simulink model "CAR_CONTROL_SYSTEM"  (R2024b)
settings: Solver=FixedStepAuto  StartTime=0.0  StopTime=inf  FixedStep=1e-3  RelTol=1e-3  EnableMultiTasking=on
model workspace (MAT data in the model file):
  SL_ROS_VariableLengthArrays_MaxSizes : object (value not decoded)
undefined symbols (not defined in the file or in its folder): angular, CIRCUIT, CLTF_DAMP, CLTF_FREQ, CLTF_GAIN, CONTROL, CONTROL_INI, DiscIntNeverNeededParam, dspblkCoreblockFVToolHelper, gcbh, INPUT, linear, MCP3201, MD25, MODEL, MODEL_INI, mpcstate, MPU60X0, MPU9250, MSG, NAV_MPC_CONTROL, OUTPUT, SAMPLING_TIME, SYSID_INPUT, VL6180X
libraries: raspberrypiCommlib x153, simulink x85, raspberrypiNetworklib x8, embedlinuxBasiclib x6, ctrlSharedLib x2, ros2lib x2, mpclib x1, vrlib x1, sldrtlib x1
(part 6 of 16)

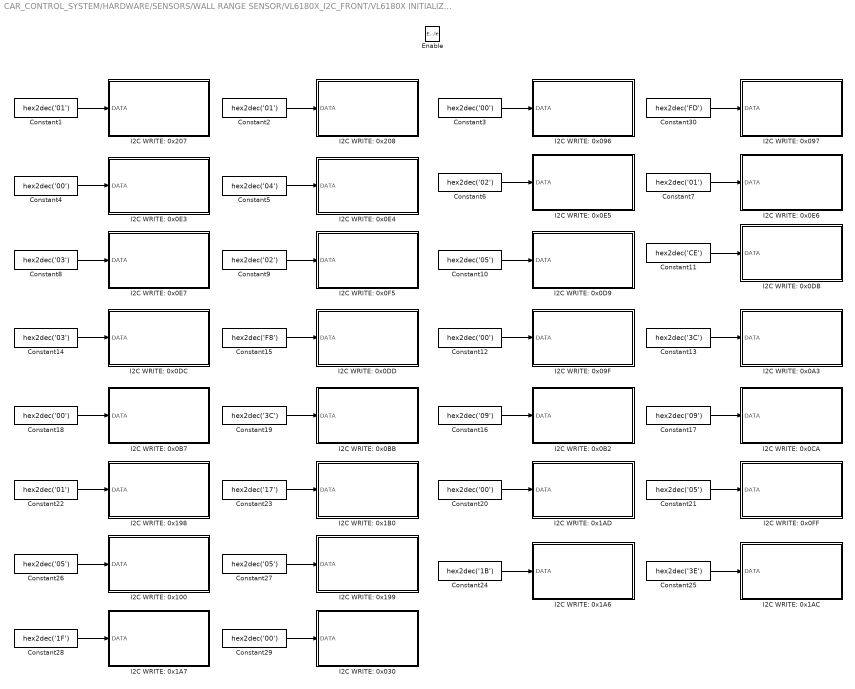
== system CAR_CONTROL_SYSTEM/HARDWARE/SENSORS/WALL RANGE SENSOR/VL6180X_I2C_FRONT/VL6180X INITIALIZATION/LOAD PRIVATE REGISTERS (MANDATORY) ==
  Enable : EnablePort
  Constant{1..2,7,22} (4 alike) : Constant  Value=hex2dec('01')  OutDataTypeStr=uint8  SampleTime=SAMPLING_TIME
  Constant{10,21,26..27} (4 alike) : Constant  Value=hex2dec('05')  OutDataTypeStr=uint8  SampleTime=SAMPLING_TIME
  Constant11 : Constant  Value=hex2dec('CE')  OutDataTypeStr=uint8  SampleTime=SAMPLING_TIME
  Constant{3..4,12,18,20,29} (6 alike) : Constant  Value=hex2dec('00')  OutDataTypeStr=uint8  SampleTime=SAMPLING_TIME
  Constant13 : Constant  Value=hex2dec('3C')  OutDataTypeStr=uint8  SampleTime=SAMPLING_TIME
  Constant14 : Constant  Value=hex2dec('03')  OutDataTypeStr=uint8  SampleTime=SAMPLING_TIME
  Constant15 : Constant  Value=hex2dec('F8')  OutDataTypeStr=uint8  SampleTime=SAMPLING_TIME
  Constant16 : Constant  Value=hex2dec('09')  OutDataTypeStr=uint8  SampleTime=SAMPLING_TIME
  Constant17 : Constant  Value=hex2dec('09')  OutDataTypeStr=uint8  SampleTime=SAMPLING_TIME
  Constant19 : Constant  Value=hex2dec('3C')  OutDataTypeStr=uint8  SampleTime=SAMPLING_TIME
  Constant23 : Constant  Value=hex2dec('17')  OutDataTypeStr=uint8  SampleTime=SAMPLING_TIME
  Constant24 : Constant  Value=hex2dec('1B')  OutDataTypeStr=uint8  SampleTime=SAMPLING_TIME
  Constant25 : Constant  Value=hex2dec('3E')  OutDataTypeStr=uint8  SampleTime=SAMPLING_TIME
  Constant28 : Constant  Value=hex2dec('1F')  OutDataTypeStr=uint8  SampleTime=SAMPLING_TIME
  Constant30 : Constant  Value=hex2dec('FD')  OutDataTypeStr=uint8  SampleTime=SAMPLING_TIME
  Constant5 : Constant  Value=hex2dec('04')  OutDataTypeStr=uint8  SampleTime=SAMPLING_TIME
  Constant6 : Constant  Value=hex2dec('02')  OutDataTypeStr=uint8  SampleTime=SAMPLING_TIME
  Constant8 : Constant  Value=hex2dec('03')  OutDataTypeStr=uint8  SampleTime=SAMPLING_TIME
  Constant9 : Constant  Value=hex2dec('02')  OutDataTypeStr=uint8  SampleTime=SAMPLING_TIME
  "I2C WRITE: 0x030 " : Subsystem  mask{SLAVE_ADDRESS=VL6180X.ADDRESS, REGISTER_ADDRESS=hex2dec('030')}
      mask prompts: SLAVE_ADDRESS "SLAVE ADDRESS"; REGISTER_ADDRESS "REGISTER ADDRESS"
      mask init:
      | REGISTER_ADDRESS_MSB = uint8(floor(REGISTER_ADDRESS/(2^8)));
      | REGISTER_ADDRESS_LSB = uint8(rem(REGISTER_ADDRESS,2^8));
  I2C WRITE: 0x096 : Subsystem  mask{SLAVE_ADDRESS=VL6180X.ADDRESS, REGISTER_ADDRESS=hex2dec('096')}
      mask prompts: SLAVE_ADDRESS "SLAVE ADDRESS"; REGISTER_ADDRESS "REGISTER ADDRESS"
      mask init:
      | REGISTER_ADDRESS_MSB = uint8(floor(REGISTER_ADDRESS/(2^8)));
      | REGISTER_ADDRESS_LSB = uint8(rem(REGISTER_ADDRESS,2^8));
  I2C WRITE: 0x097 : Subsystem  mask{SLAVE_ADDRESS=VL6180X.ADDRESS, REGISTER_ADDRESS=hex2dec('097')}
      mask prompts: SLAVE_ADDRESS "SLAVE ADDRESS"; REGISTER_ADDRESS "REGISTER ADDRESS"
      mask init:
      | REGISTER_ADDRESS_MSB = uint8(floor(REGISTER_ADDRESS/(2^8)));
      | REGISTER_ADDRESS_LSB = uint8(rem(REGISTER_ADDRESS,2^8));
  I2C WRITE: 0x09F : Subsystem  mask{SLAVE_ADDRESS=VL6180X.ADDRESS, REGISTER_ADDRESS=hex2dec('09F')}
      mask prompts: SLAVE_ADDRESS "SLAVE ADDRESS"; REGISTER_ADDRESS "REGISTER ADDRESS"
      mask init:
      | REGISTER_ADDRESS_MSB = uint8(floor(REGISTER_ADDRESS/(2^8)));
      | REGISTER_ADDRESS_LSB = uint8(rem(REGISTER_ADDRESS,2^8));
  I2C WRITE: 0x0A3 : Subsystem  mask{SLAVE_ADDRESS=VL6180X.ADDRESS, REGISTER_ADDRESS=hex2dec('0A3')}
      mask prompts: SLAVE_ADDRESS "SLAVE ADDRESS"; REGISTER_ADDRESS "REGISTER ADDRESS"
      mask init:
      | REGISTER_ADDRESS_MSB = uint8(floor(REGISTER_ADDRESS/(2^8)));
      | REGISTER_ADDRESS_LSB = uint8(rem(REGISTER_ADDRESS,2^8));
  I2C WRITE: 0x0B2 : Subsystem  mask{SLAVE_ADDRESS=VL6180X.ADDRESS, REGISTER_ADDRESS=hex2dec('0B2')}
      mask prompts: SLAVE_ADDRESS "SLAVE ADDRESS"; REGISTER_ADDRESS "REGISTER ADDRESS"
      mask init:
      | REGISTER_ADDRESS_MSB = uint8(floor(REGISTER_ADDRESS/(2^8)));
      | REGISTER_ADDRESS_LSB = uint8(rem(REGISTER_ADDRESS,2^8));
  I2C WRITE: 0x0B7 : Subsystem  mask{SLAVE_ADDRESS=VL6180X.ADDRESS, REGISTER_ADDRESS=hex2dec('0B7')}
      mask prompts: SLAVE_ADDRESS "SLAVE ADDRESS"; REGISTER_ADDRESS "REGISTER ADDRESS"
      mask init:
      | REGISTER_ADDRESS_MSB = uint8(floor(REGISTER_ADDRESS/(2^8)));
      | REGISTER_ADDRESS_LSB = uint8(rem(REGISTER_ADDRESS,2^8));
  I2C WRITE: 0x0BB : Subsystem  mask{SLAVE_ADDRESS=VL6180X.ADDRESS, REGISTER_ADDRESS=hex2dec('0BB')}
      mask prompts: SLAVE_ADDRESS "SLAVE ADDRESS"; REGISTER_ADDRESS "REGISTER ADDRESS"
      mask init:
      | REGISTER_ADDRESS_MSB = uint8(floor(REGISTER_ADDRESS/(2^8)));
      | REGISTER_ADDRESS_LSB = uint8(rem(REGISTER_ADDRESS,2^8));
  I2C WRITE: 0x0CA : Subsystem  mask{SLAVE_ADDRESS=VL6180X.ADDRESS, REGISTER_ADDRESS=hex2dec('0CA')}
      mask prompts: SLAVE_ADDRESS "SLAVE ADDRESS"; REGISTER_ADDRESS "REGISTER ADDRESS"
      mask init:
      | REGISTER_ADDRESS_MSB = uint8(floor(REGISTER_ADDRESS/(2^8)));
      | REGISTER_ADDRESS_LSB = uint8(rem(REGISTER_ADDRESS,2^8));
  I2C WRITE: 0x0D9 : Subsystem  mask{SLAVE_ADDRESS=VL6180X.ADDRESS, REGISTER_ADDRESS=hex2dec('0D9')}
      mask prompts: SLAVE_ADDRESS "SLAVE ADDRESS"; REGISTER_ADDRESS "REGISTER ADDRESS"
      mask init:
      | REGISTER_ADDRESS_MSB = uint8(floor(REGISTER_ADDRESS/(2^8)));
      | REGISTER_ADDRESS_LSB = uint8(rem(REGISTER_ADDRESS,2^8));
  I2C WRITE: 0x0DB : Subsystem  mask{SLAVE_ADDRESS=VL6180X.ADDRESS, REGISTER_ADDRESS=hex2dec('0DB')}
      mask prompts: SLAVE_ADDRESS "SLAVE ADDRESS"; REGISTER_ADDRESS "REGISTER ADDRESS"
      mask init:
      | REGISTER_ADDRESS_MSB = uint8(floor(REGISTER_ADDRESS/(2^8)));
      | REGISTER_ADDRESS_LSB = uint8(rem(REGISTER_ADDRESS,2^8));
  I2C WRITE: 0x0DC : Subsystem  mask{SLAVE_ADDRESS=VL6180X.ADDRESS, REGISTER_ADDRESS=hex2dec('0DB')}
      mask prompts: SLAVE_ADDRESS "SLAVE ADDRESS"; REGISTER_ADDRESS "REGISTER ADDRESS"
      mask init:
      | REGISTER_ADDRESS_MSB = uint8(floor(REGISTER_ADDRESS/(2^8)));
      | REGISTER_ADDRESS_LSB = uint8(rem(REGISTER_ADDRESS,2^8));
  I2C WRITE: 0x0DD : Subsystem  mask{SLAVE_ADDRESS=VL6180X.ADDRESS, REGISTER_ADDRESS=hex2dec('0DD')}
      mask prompts: SLAVE_ADDRESS "SLAVE ADDRESS"; REGISTER_ADDRESS "REGISTER ADDRESS"
      mask init:
      | REGISTER_ADDRESS_MSB = uint8(floor(REGISTER_ADDRESS/(2^8)));
      | REGISTER_ADDRESS_LSB = uint8(rem(REGISTER_ADDRESS,2^8));
  I2C WRITE: 0x0E3 : Subsystem  mask{SLAVE_ADDRESS=VL6180X.ADDRESS, REGISTER_ADDRESS=hex2dec('0E3')}
      mask prompts: SLAVE_ADDRESS "SLAVE ADDRESS"; REGISTER_ADDRESS "REGISTER ADDRESS"
      mask init:
      | REGISTER_ADDRESS_MSB = uint8(floor(REGISTER_ADDRESS/(2^8)));
      | REGISTER_ADDRESS_LSB = uint8(rem(REGISTER_ADDRESS,2^8));
  I2C WRITE: 0x0E4 : Subsystem  mask{SLAVE_ADDRESS=VL6180X.ADDRESS, REGISTER_ADDRESS=hex2dec('0E4')}
      mask prompts: SLAVE_ADDRESS "SLAVE ADDRESS"; REGISTER_ADDRESS "REGISTER ADDRESS"
      mask init:
      | REGISTER_ADDRESS_MSB = uint8(floor(REGISTER_ADDRESS/(2^8)));
      | REGISTER_ADDRESS_LSB = uint8(rem(REGISTER_ADDRESS,2^8));
  I2C WRITE: 0x0E5 : Subsystem  mask{SLAVE_ADDRESS=VL6180X.ADDRESS, REGISTER_ADDRESS=hex2dec('0E5')}
      mask prompts: SLAVE_ADDRESS "SLAVE ADDRESS"; REGISTER_ADDRESS "REGISTER ADDRESS"
      mask init:
      | REGISTER_ADDRESS_MSB = uint8(floor(REGISTER_ADDRESS/(2^8)));
      | REGISTER_ADDRESS_LSB = uint8(rem(REGISTER_ADDRESS,2^8));
  I2C WRITE: 0x0E6 : Subsystem  mask{SLAVE_ADDRESS=VL6180X.ADDRESS, REGISTER_ADDRESS=hex2dec('0E6')}
      mask prompts: SLAVE_ADDRESS "SLAVE ADDRESS"; REGISTER_ADDRESS "REGISTER ADDRESS"
      mask init:
      | REGISTER_ADDRESS_MSB = uint8(floor(REGISTER_ADDRESS/(2^8)));
      | REGISTER_ADDRESS_LSB = uint8(rem(REGISTER_ADDRESS,2^8));
  I2C WRITE: 0x0E7 : Subsystem  mask{SLAVE_ADDRESS=VL6180X.ADDRESS, REGISTER_ADDRESS=hex2dec('0E7')}
      mask prompts: SLAVE_ADDRESS "SLAVE ADDRESS"; REGISTER_ADDRESS "REGISTER ADDRESS"
      mask init:
      | REGISTER_ADDRESS_MSB = uint8(floor(REGISTER_ADDRESS/(2^8)));
      | REGISTER_ADDRESS_LSB = uint8(rem(REGISTER_ADDRESS,2^8));
  I2C WRITE: 0x0F5 : Subsystem  mask{SLAVE_ADDRESS=VL6180X.ADDRESS, REGISTER_ADDRESS=hex2dec('0F5')}
      mask prompts: SLAVE_ADDRESS "SLAVE ADDRESS"; REGISTER_ADDRESS "REGISTER ADDRESS"
      mask init:
      | REGISTER_ADDRESS_MSB = uint8(floor(REGISTER_ADDRESS/(2^8)));
      | REGISTER_ADDRESS_LSB = uint8(rem(REGISTER_ADDRESS,2^8));
  "I2C WRITE: 0x0FF " : Subsystem  mask{SLAVE_ADDRESS=VL6180X.ADDRESS, REGISTER_ADDRESS=hex2dec('0FF')}
      mask prompts: SLAVE_ADDRESS "SLAVE ADDRESS"; REGISTER_ADDRESS "REGISTER ADDRESS"
      mask init:
      | REGISTER_ADDRESS_MSB = uint8(floor(REGISTER_ADDRESS/(2^8)));
      | REGISTER_ADDRESS_LSB = uint8(rem(REGISTER_ADDRESS,2^8));
  "I2C WRITE: 0x100 " : Subsystem  mask{SLAVE_ADDRESS=VL6180X.ADDRESS, REGISTER_ADDRESS=hex2dec('100')}
      mask prompts: SLAVE_ADDRESS "SLAVE ADDRESS"; REGISTER_ADDRESS "REGISTER ADDRESS"
      mask init:
      | REGISTER_ADDRESS_MSB = uint8(floor(REGISTER_ADDRESS/(2^8)));
      | REGISTER_ADDRESS_LSB = uint8(rem(REGISTER_ADDRESS,2^8));
  I2C WRITE: 0x198 : Subsystem  mask{SLAVE_ADDRESS=VL6180X.ADDRESS, REGISTER_ADDRESS=hex2dec('198')}
      mask prompts: SLAVE_ADDRESS "SLAVE ADDRESS"; REGISTER_ADDRESS "REGISTER ADDRESS"
      mask init:
      | REGISTER_ADDRESS_MSB = uint8(floor(REGISTER_ADDRESS/(2^8)));
      | REGISTER_ADDRESS_LSB = uint8(rem(REGISTER_ADDRESS,2^8));
  "I2C WRITE: 0x199 " : Subsystem  mask{SLAVE_ADDRESS=VL6180X.ADDRESS, REGISTER_ADDRESS=hex2dec('199')}
      mask prompts: SLAVE_ADDRESS "SLAVE ADDRESS"; REGISTER_ADDRESS "REGISTER ADDRESS"
      mask init:
      | REGISTER_ADDRESS_MSB = uint8(floor(REGISTER_ADDRESS/(2^8)));
      | REGISTER_ADDRESS_LSB = uint8(rem(REGISTER_ADDRESS,2^8));
  "I2C WRITE: 0x1A6 " : Subsystem  mask{SLAVE_ADDRESS=VL6180X.ADDRESS, REGISTER_ADDRESS=hex2dec('1A6')}
      mask prompts: SLAVE_ADDRESS "SLAVE ADDRESS"; REGISTER_ADDRESS "REGISTER ADDRESS"
      mask init:
      | REGISTER_ADDRESS_MSB = uint8(floor(REGISTER_ADDRESS/(2^8)));
      | REGISTER_ADDRESS_LSB = uint8(rem(REGISTER_ADDRESS,2^8));
  "I2C WRITE: 0x1A7 " : Subsystem  mask{SLAVE_ADDRESS=VL6180X.ADDRESS, REGISTER_ADDRESS=hex2dec('1A7')}
      mask prompts: SLAVE_ADDRESS "SLAVE ADDRESS"; REGISTER_ADDRESS "REGISTER ADDRESS"
      mask init:
      | REGISTER_ADDRESS_MSB = uint8(floor(REGISTER_ADDRESS/(2^8)));
      | REGISTER_ADDRESS_LSB = uint8(rem(REGISTER_ADDRESS,2^8));
  "I2C WRITE: 0x1AC " : Subsystem  mask{SLAVE_ADDRESS=VL6180X.ADDRESS, REGISTER_ADDRESS=hex2dec('1AC')}
      mask prompts: SLAVE_ADDRESS "SLAVE ADDRESS"; REGISTER_ADDRESS "REGISTER ADDRESS"
      mask init:
      | REGISTER_ADDRESS_MSB = uint8(floor(REGISTER_ADDRESS/(2^8)));
      | REGISTER_ADDRESS_LSB = uint8(rem(REGISTER_ADDRESS,2^8));
  "I2C WRITE: 0x1AD " : Subsystem  mask{SLAVE_ADDRESS=VL6180X.ADDRESS, REGISTER_ADDRESS=hex2dec('1AD')}
      mask prompts: SLAVE_ADDRESS "SLAVE ADDRESS"; REGISTER_ADDRESS "REGISTER ADDRESS"
      mask init:
      | REGISTER_ADDRESS_MSB = uint8(floor(REGISTER_ADDRESS/(2^8)));
      | REGISTER_ADDRESS_LSB = uint8(rem(REGISTER_ADDRESS,2^8));
  "I2C WRITE: 0x1B0 " : Subsystem  mask{SLAVE_ADDRESS=VL6180X.ADDRESS, REGISTER_ADDRESS=hex2dec('1B0')}
      mask prompts: SLAVE_ADDRESS "SLAVE ADDRESS"; REGISTER_ADDRESS "REGISTER ADDRESS"
      mask init:
      | REGISTER_ADDRESS_MSB = uint8(floor(REGISTER_ADDRESS/(2^8)));
      | REGISTER_ADDRESS_LSB = uint8(rem(REGISTER_ADDRESS,2^8));
  I2C WRITE: 0x207 : Subsystem  mask{SLAVE_ADDRESS=VL6180X.ADDRESS, REGISTER_ADDRESS=hex2dec('207')}
      mask prompts: SLAVE_ADDRESS "SLAVE ADDRESS"; REGISTER_ADDRESS "REGISTER ADDRESS"
      mask init:
      | REGISTER_ADDRESS_MSB = uint8(floor(REGISTER_ADDRESS/(2^8)));
      | REGISTER_ADDRESS_LSB = uint8(rem(REGISTER_ADDRESS,2^8));
  I2C WRITE: 0x208 : Subsystem  mask{SLAVE_ADDRESS=VL6180X.ADDRESS, REGISTER_ADDRESS=hex2dec('208')}
      mask prompts: SLAVE_ADDRESS "SLAVE ADDRESS"; REGISTER_ADDRESS "REGISTER ADDRESS"
      mask init:
      | REGISTER_ADDRESS_MSB = uint8(floor(REGISTER_ADDRESS/(2^8)));
      | REGISTER_ADDRESS_LSB = uint8(rem(REGISTER_ADDRESS,2^8));
  wires:
  Constant1/1 -> I2C WRITE: 0x207/1(DATA)
  Constant2/1 -> I2C WRITE: 0x208/1(DATA)
  Constant3/1 -> I2C WRITE: 0x096/1(DATA)
  Constant30/1 -> I2C WRITE: 0x097/1(DATA)
  Constant4/1 -> I2C WRITE: 0x0E3/1(DATA)
  Constant5/1 -> I2C WRITE: 0x0E4/1(DATA)
  Constant6/1 -> I2C WRITE: 0x0E5/1(DATA)
  Constant7/1 -> I2C WRITE: 0x0E6/1(DATA)
  Constant8/1 -> I2C WRITE: 0x0E7/1(DATA)
  Constant9/1 -> I2C WRITE: 0x0F5/1(DATA)
  Constant10/1 -> I2C WRITE: 0x0D9/1(DATA)
  Constant11/1 -> I2C WRITE: 0x0DB/1(DATA)
  Constant14/1 -> I2C WRITE: 0x0DC/1(DATA)
  Constant15/1 -> I2C WRITE: 0x0DD/1(DATA)
  Constant12/1 -> I2C WRITE: 0x09F/1(DATA)
  Constant13/1 -> I2C WRITE: 0x0A3/1(DATA)
  Constant18/1 -> I2C WRITE: 0x0B7/1(DATA)
  Constant19/1 -> I2C WRITE: 0x0BB/1(DATA)
  Constant16/1 -> I2C WRITE: 0x0B2/1(DATA)
  Constant17/1 -> I2C WRITE: 0x0CA/1(DATA)
  Constant22/1 -> I2C WRITE: 0x198/1(DATA)
  Constant23/1 -> "I2C WRITE: 0x1B0 "/1(DATA)
  Constant20/1 -> "I2C WRITE: 0x1AD "/1(DATA)
  Constant21/1 -> "I2C WRITE: 0x0FF "/1(DATA)
  Constant26/1 -> "I2C WRITE: 0x100 "/1(DATA)
  Constant27/1 -> "I2C WRITE: 0x199 "/1(DATA)
  Constant24/1 -> "I2C WRITE: 0x1A6 "/1(DATA)
  Constant25/1 -> "I2C WRITE: 0x1AC "/1(DATA)
  Constant28/1 -> "I2C WRITE: 0x1A7 "/1(DATA)
  Constant29/1 -> "I2C WRITE: 0x030 "/1(DATA)

== system CAR_CONTROL_SYSTEM/HARDWARE/SENSORS/WALL RANGE SENSOR/VL6180X_I2C_FRONT/VL6180X INITIALIZATION/LOAD PUBLIC REGISTERS (OPTIONAL) ==
  note: als_int_mode = 4 (ALS new sample ready interrupt);
      | range_int_mode = 4 (range new sample ready interrupt)
  note: sysals__intermeasurement_period = 49 (500 ms)
  note: sysrange__intermeasurement_period = 1 (20 ms)
  Enable : EnablePort
  Constant2 : Constant  Value=VL6180X.SYSRANGE_INTERMEASUREMENT_PERIOD_BYTE  OutDataTypeStr=uint8  SampleTime=SAMPLING_TIME
  Constant3 : Constant  Value=hex2dec('24')  OutDataTypeStr=uint8  SampleTime=SAMPLING_TIME
  Constant4 : Constant  Commented=on  Value=VL6180X.SYSALS_INTERMEASUREMENT_PERIOD_BYTE  OutDataTypeStr=uint8  SampleTime=SAMPLING_TIME
  I2C WRITE: SYSRANGE_INTERMEASUREMENT_PERIOD : Subsystem  mask{SLAVE_ADDRESS=VL6180X.ADDRESS, REGISTER_ADDRESS=VL6180X.SYSRANGE_INTERMEASUREMENT_PERIOD}
      mask prompts: SLAVE_ADDRESS "SLAVE ADDRESS"; REGISTER_ADDRESS "REGISTER ADDRESS"
      mask init:
      | REGISTER_ADDRESS_MSB = uint8(floor(REGISTER_ADDRESS/(2^8)));
      | REGISTER_ADDRESS_LSB = uint8(rem(REGISTER_ADDRESS,2^8));
  I2C WRITE: SYSALS_INTERMEASUREMENT_PERIOD : Subsystem  Commented=on  mask{SLAVE_ADDRESS=VL6180X.ADDRESS, REGISTER_ADDRESS=VL6180X.SYSALS_INTERMEASUREMENT_PERIOD}
      mask prompts: SLAVE_ADDRESS "SLAVE ADDRESS"; REGISTER_ADDRESS "REGISTER ADDRESS"
      mask init:
      | REGISTER_ADDRESS_MSB = uint8(floor(REGISTER_ADDRESS/(2^8)));
      | REGISTER_ADDRESS_LSB = uint8(rem(REGISTER_ADDRESS,2^8));
  I2C WRITE: SYSTEM_INTERRUPT_CONFIG_GPIO : Subsystem  mask{SLAVE_ADDRESS=VL6180X.ADDRESS, REGISTER_ADDRESS=VL6180X.SYSTEM_INTERRUPT_CONFIG_GPIO}
      mask prompts: SLAVE_ADDRESS "SLAVE ADDRESS"; REGISTER_ADDRESS "REGISTER ADDRESS"
      mask init:
      | REGISTER_ADDRESS_MSB = uint8(floor(REGISTER_ADDRESS/(2^8)));
      | REGISTER_ADDRESS_LSB = uint8(rem(REGISTER_ADDRESS,2^8));
  wires:
  Constant4/1 -> I2C WRITE: SYSALS_INTERMEASUREMENT_PERIOD/1(DATA)
  Constant3/1 -> I2C WRITE: SYSTEM_INTERRUPT_CONFIG_GPIO/1(DATA)
  Constant2/1 -> I2C WRITE: SYSRANGE_INTERMEASUREMENT_PERIOD/1(DATA)

== system CAR_CONTROL_SYSTEM/HARDWARE/SENSORS/WALL RANGE SENSOR/VL6180X_I2C_FRONT/VL6180X INITIALIZATION/LOAD PUBLIC REGISTERS (RECOMMENDED) ==
  note: set up GPIO1 as an interrupt output as suggested,
      | though you can do so by calling:
  note: readout__averaging_sample_period = 48
  note: sysals__analogue_gain_light = 6
      | (ALS gain = 1 nominal, actually 1.01 according to Table 14 in datasheet)
  note: sysrange__vhv_repeat_rate = 255
      | (auto Very High Voltage temperature recalibration after every 255 range measurements)
  note: sysals__integration_period = 99 (100 ms)
      | AN4545 incorrectly recommends writing to register 0x040;
      | 0x63 should go in the lower byte, which is register 0x041.
  note: sysrange__vhv_recalibrate = 1 (manually trigger a VHV recalibration)
  Enable : EnablePort
  Constant1 : Constant  Value=hex2dec('10')  OutDataTypeStr=uint8  SampleTime=SAMPLING_TIME
  Constant2 : Constant  Value=hex2dec('30')  OutDataTypeStr=uint8  SampleTime=SAMPLING_TIME
  Constant3 : Constant  Value=hex2dec('46')  OutDataTypeStr=uint8  SampleTime=SAMPLING_TIME
  Constant4 : Constant  Value=hex2dec('FF')  OutDataTypeStr=uint8  SampleTime=SAMPLING_TIME
  Constant5 : Constant  Value=hex2dec('63')  OutDataTypeStr=uint8  SampleTime=SAMPLING_TIME
  Constant6 : Constant  Value=hex2dec('01')  OutDataTypeStr=uint8  SampleTime=SAMPLING_TIME
  Constant7 : Constant  Value=hex2dec('00')  OutDataTypeStr=uint8  SampleTime=SAMPLING_TIME
  I2C WRITE: READOUT_AVERAGING_SAMPLE_PERIOD : Subsystem  mask{SLAVE_ADDRESS=VL6180X.ADDRESS, REGISTER_ADDRESS=VL6180X.READOUT_AVERAGING_SAMPLE_PERIOD}
      mask prompts: SLAVE_ADDRESS "SLAVE ADDRESS"; REGISTER_ADDRESS "REGISTER ADDRESS"
      mask init:
      | REGISTER_ADDRESS_MSB = uint8(floor(REGISTER_ADDRESS/(2^8)));
      | REGISTER_ADDRESS_LSB = uint8(rem(REGISTER_ADDRESS,2^8));
  I2C WRITE: SYSALS_ANALOGUE_GAIN : Subsystem  mask{SLAVE_ADDRESS=VL6180X.ADDRESS, REGISTER_ADDRESS=VL6180X.SYSALS_ANALOGUE_GAIN}
      mask prompts: SLAVE_ADDRESS "SLAVE ADDRESS"; REGISTER_ADDRESS "REGISTER ADDRESS"
      mask init:
      | REGISTER_ADDRESS_MSB = uint8(floor(REGISTER_ADDRESS/(2^8)));
      | REGISTER_ADDRESS_LSB = uint8(rem(REGISTER_ADDRESS,2^8));
  I2C WRITE: SYSALS_INTEGRATION_PERIOD : Subsystem  mask{SLAVE_ADDRESS=VL6180X.ADDRESS, REGISTER_ADDRESS=VL6180X.SYSALS_INTEGRATION_PERIOD}
      mask prompts: SLAVE_ADDRESS "SLAVE ADDRESS"; REGISTER_ADDRESS "REGISTER ADDRESS"
      mask init:
      | REGISTER_ADDRESS_MSB = uint8(floor(REGISTER_ADDRESS/(2^8)));
      | REGISTER_ADDRESS_LSB = uint8(rem(REGISTER_ADDRESS,2^8));
  I2C WRITE: SYSRANGE_VHV_RECALIBRATE : Subsystem  mask{SLAVE_ADDRESS=VL6180X.ADDRESS, REGISTER_ADDRESS=VL6180X.SYSRANGE_VHV_RECALIBRATE}
      mask prompts: SLAVE_ADDRESS "SLAVE ADDRESS"; REGISTER_ADDRESS "REGISTER ADDRESS"
      mask init:
      | REGISTER_ADDRESS_MSB = uint8(floor(REGISTER_ADDRESS/(2^8)));
      | REGISTER_ADDRESS_LSB = uint8(rem(REGISTER_ADDRESS,2^8));
  I2C WRITE: SYSRANGE_VHV_REPEAT_RATE : Subsystem  mask{SLAVE_ADDRESS=VL6180X.ADDRESS, REGISTER_ADDRESS=VL6180X.SYSRANGE_VHV_REPEAT_RATE}
      mask prompts: SLAVE_ADDRESS "SLAVE ADDRESS"; REGISTER_ADDRESS "REGISTER ADDRESS"
      mask init:
      | REGISTER_ADDRESS_MSB = uint8(floor(REGISTER_ADDRESS/(2^8)));
      | REGISTER_ADDRESS_LSB = uint8(rem(REGISTER_ADDRESS,2^8));
  I2C WRITE: SYSTEM_MODE_GPIO1 : Subsystem  mask{SLAVE_ADDRESS=VL6180X.ADDRESS, REGISTER_ADDRESS=VL6180X.SYSTEM_MODE_GPIO1}
      mask prompts: SLAVE_ADDRESS "SLAVE ADDRESS"; REGISTER_ADDRESS "REGISTER ADDRESS"
      mask init:
      | REGISTER_ADDRESS_MSB = uint8(floor(REGISTER_ADDRESS/(2^8)));
      | REGISTER_ADDRESS_LSB = uint8(rem(REGISTER_ADDRESS,2^8));
  Mux : Mux  Inputs=2
  wires:
  Constant1/1 -> I2C WRITE: SYSTEM_MODE_GPIO1/1(DATA)
  Constant2/1 -> I2C WRITE: READOUT_AVERAGING_SAMPLE_PERIOD/1(DATA)
  Constant3/1 -> I2C WRITE: SYSALS_ANALOGUE_GAIN/1(DATA)
  Constant4/1 -> I2C WRITE: SYSRANGE_VHV_REPEAT_RATE/1(DATA)
  Mux/1 -> I2C WRITE: SYSALS_INTEGRATION_PERIOD/1(DATA)
  Constant5/1 -> Mux/2
  Constant7/1 -> Mux/1
  Constant6/1 -> I2C WRITE: SYSRANGE_VHV_RECALIBRATE/1(DATA)

== system CAR_CONTROL_SYSTEM/HARDWARE/SENSORS/WALL RANGE SENSOR/VL6180X_I2C_FRONT/VL6180X INITIALIZATION/MEASUREMENT CONFIGURATION ==
  Enable : EnablePort
  CONTINUOUS : simulink/Logic and Bit Operations/Compare To Constant  relop===  const=1  OutDataTypeStr=boolean
  Constant1 : Constant  Value=hex2dec('07')  OutDataTypeStr=uint8  SampleTime=SAMPLING_TIME
  Data Store Write1 : DataStoreWrite  Priority=100  DataStoreName=VL6180X_STATUS  IndexOptions=Index vector (dialog)  Indices=1  OutputSizes=1
  I2C WRITE: SYSTEM_INTERRUPT_CLEAR : Subsystem  Priority=5  mask{SLAVE_ADDRESS=VL6180X.ADDRESS, REGISTER_ADDRESS=VL6180X.SYSTEM_INTERRUPT_CLEAR}
      mask prompts: SLAVE_ADDRESS "SLAVE ADDRESS"; REGISTER_ADDRESS "REGISTER ADDRESS"
      mask init:
      | REGISTER_ADDRESS_MSB = uint8(floor(REGISTER_ADDRESS/(2^8)));
      | REGISTER_ADDRESS_LSB = uint8(rem(REGISTER_ADDRESS,2^8));
  MEASUREMENT : Constant  OutDataTypeStr=uint8  SampleTime=SAMPLING_TIME
  READY1 : Constant  Value=VL6180X.RANGING_MODE  OutDataTypeStr=uint8  SampleTime=SAMPLING_TIME
  SINGLE_SHOT : simulink/Logic and Bit Operations/Compare To Constant  relop===  const=0  OutDataTypeStr=boolean
  START READ RANGE CONTINUOUS : Subsystem  Priority=20  TreatAsAtomicUnit=on
      settings: RTWSystemCode=Nonreusable function
  START READ RANGE SINGLE : Subsystem  Priority=10  TreatAsAtomicUnit=on
      settings: RTWSystemCode=Nonreusable function
  wires:
  MEASUREMENT/1 -> Data Store Write1/1
  READY1/1 -> CONTINUOUS/1, SINGLE_SHOT/1
  SINGLE_SHOT/1 -> START READ RANGE SINGLE/Enable
  CONTINUOUS/1 -> START READ RANGE CONTINUOUS/Enable
  Constant1/1 -> I2C WRITE: SYSTEM_INTERRUPT_CLEAR/1(DATA)

== system CAR_CONTROL_SYSTEM/HARDWARE/SENSORS/WALL RANGE SENSOR/VL6180X_I2C_FRONT/VL6180X INITIALIZATION/OTHER SPECIFIC SETTINGS (OPTIONAL) ==
  note: RESET OTHER SETTINGS TO POWER-ON DEFAULTS
  note: sysrange_max_convergence_time = 49 (49 ms)
  note: disable interleaved mode
  Enable : EnablePort
  Constant1 : Constant  Value=hex2dec('00')  OutDataTypeStr=uint8  SampleTime=SAMPLING_TIME
  Constant2 : Constant  Value=hex2dec('31')  OutDataTypeStr=uint8  SampleTime=SAMPLING_TIME
  I2C WRITE: INTERLEAVED_MODE_ENABLE : Subsystem  mask{SLAVE_ADDRESS=VL6180X.ADDRESS, REGISTER_ADDRESS=VL6180X.INTERLEAVED_MODE_ENABLE}
      mask prompts: SLAVE_ADDRESS "SLAVE ADDRESS"; REGISTER_ADDRESS "REGISTER ADDRESS"
      mask init:
      | REGISTER_ADDRESS_MSB = uint8(floor(REGISTER_ADDRESS/(2^8)));
      | REGISTER_ADDRESS_LSB = uint8(rem(REGISTER_ADDRESS,2^8));
  I2C WRITE: SYSRANGE_MAX_CONVERGENCE_TIME : Subsystem  mask{SLAVE_ADDRESS=VL6180X.ADDRESS, REGISTER_ADDRESS=VL6180X.SYSRANGE_MAX_CONVERGENCE_TIME}
      mask prompts: SLAVE_ADDRESS "SLAVE ADDRESS"; REGISTER_ADDRESS "REGISTER ADDRESS"
      mask init:
      | REGISTER_ADDRESS_MSB = uint8(floor(REGISTER_ADDRESS/(2^8)));
      | REGISTER_ADDRESS_LSB = uint8(rem(REGISTER_ADDRESS,2^8));
  wires:
  Constant2/1 -> I2C WRITE: SYSRANGE_MAX_CONVERGENCE_TIME/1(DATA)
  Constant1/1 -> I2C WRITE: INTERLEAVED_MODE_ENABLE/1(DATA)

== system CAR_CONTROL_SYSTEM/HARDWARE/SENSORS/WALL RANGE SENSOR/VL6180X_I2C_REAR/READ RANGE/CHECK READOUT ==
  Enable : EnablePort
  Bias : Bias  Bias=1  SaturateOnIntegerOverflow=off
  Compare To Constant : simulink/Logic and Bit Operations/Compare To Constant  relop=>=  const=20  OutDataTypeStr=boolean
  Data Store Read1 : DataStoreRead  DataStoreName=VL6180X_COUNTER  SampleTime=SAMPLING_TIME  IndexOptions=Index vector (dialog)  Indices=1  OutputSizes=1
  Data Store Write : DataStoreWrite  DataStoreName=VL6180X_COUNTER  IndexOptions=Index vector (dialog)  Indices=1  OutputSizes=1
  SENSOR INITIALIZATION : Subsystem
  wires:
  Compare To Constant/1 -> SENSOR INITIALIZATION/Enable
  Bias/1 -> Data Store Write/1, Compare To Constant/1
  Data Store Read1/1 -> Bias/1

== system CAR_CONTROL_SYSTEM/HARDWARE/SENSORS/WALL RANGE SENSOR/VL6180X_I2C_REAR/READ RANGE/I2C READ: RESULT_INTERRUPT_STATUS_GPIO ==
  Constant : Constant  Value=REGISTER_ADDRESS  OutDataTypeStr=uint16  SampleTime=SAMPLING_TIME
  DATA TO BE READ : raspberrypiCommlib/I2C Controller Read  Priority=20  BoardProperty=Pi 3 Model B  I2CModule=1  Mode=Master  SlaveAddress=SLAVE_ADDRESS  SlaveByteOrder=BigEndian  Direction=Receiver  RegisterAddressMode=off  RegisterAddress=0  SlaveDataType=uint8  DataLength=uint8(N)  NoAck=off  RepeatedStart=off  OutputStatus=off  SampleTime=SAMPLING_TIME
  REGISTER ADDRESS : raspberrypiCommlib/I2C Controller Write  Priority=10  BoardProperty=Pi 3 Model B  I2CModule=1  Mode=Master  SlaveAddress=SLAVE_ADDRESS  SlaveByteOrder=BigEndian  Direction=Transmitter  RegisterAddressMode=off  RegisterAddress=hex2dec('207')  SlaveDataType=uint8  DataLength=1  NoAck=off  RepeatedStart=off  OutputStatus=off
  DATA : Outport  VectorParamsAs1DForOutWhenUnconnected=off
  wires:
  Constant/1 -> REGISTER ADDRESS/1
  DATA TO BE READ/1 -> DATA/1

== system CAR_CONTROL_SYSTEM/HARDWARE/SENSORS/WALL RANGE SENSOR/VL6180X_I2C_REAR/READ RANGE/READ RANGE VALUE ==
  Enable : EnablePort
  Constant1 : Constant  Value=hex2dec('07')  OutDataTypeStr=uint8  SampleTime=SAMPLING_TIME
  Data Store Write : DataStoreWrite  DataStoreName=VL6180X_RANGE_VAL  IndexOptions=Index vector (dialog)  Indices=1  OutputSizes=1
  Data Store Write1 : DataStoreWrite  DataStoreName=VL6180X_COUNTER  IndexOptions=Index vector (dialog)  Indices=1  OutputSizes=1
  I2C READ: VL6180X.RESULT_RANGE_VAL : Subsystem  Priority=10  mask{SLAVE_ADDRESS=VL6180X.ADDRESS, REGISTER_ADDRESS=VL6180X.RESULT_RANGE_VAL, N=1}
      mask prompts: SLAVE_ADDRESS "SLAVE ADDRESS"; REGISTER_ADDRESS "REGISTER ADDRESS"; N "NUMBER OF DATA (bytes)"
  I2C WRITE: SYSTEM_INTERRUPT_CLEAR : Subsystem  Priority=20  mask{SLAVE_ADDRESS=VL6180X.ADDRESS, REGISTER_ADDRESS=VL6180X.SYSTEM_INTERRUPT_CLEAR}
      mask prompts: SLAVE_ADDRESS "SLAVE ADDRESS"; REGISTER_ADDRESS "REGISTER ADDRESS"
      mask init:
      | REGISTER_ADDRESS_MSB = uint8(floor(REGISTER_ADDRESS/(2^8)));
      | REGISTER_ADDRESS_LSB = uint8(rem(REGISTER_ADDRESS,2^8));
  READY1 : Constant  Value=0  OutDataTypeStr=uint8  SampleTime=SAMPLING_TIME
  wires:
  READY1/1 -> Data Store Write1/1
  Constant1/1 -> I2C WRITE: SYSTEM_INTERRUPT_CLEAR/1(DATA)
  I2C READ: VL6180X.RESULT_RANGE_VAL/1(DATA) -> Data Store Write/1

== system CAR_CONTROL_SYSTEM/HARDWARE/SENSORS/WALL RANGE SENSOR/VL6180X_I2C_REAR/READ RANGE/START READ RANGE SINGLE ==
  Enable : EnablePort
  Constant1 : Constant  Value=hex2dec('01')  OutDataTypeStr=uint8  SampleTime=SAMPLING_TIME
  I2C WRITE: SYSRANGE_START : Subsystem  mask{SLAVE_ADDRESS=VL6180X.ADDRESS, REGISTER_ADDRESS=VL6180X.SYSRANGE_START}
      mask prompts: SLAVE_ADDRESS "SLAVE ADDRESS"; REGISTER_ADDRESS "REGISTER ADDRESS"
      mask init:
      | REGISTER_ADDRESS_MSB = uint8(floor(REGISTER_ADDRESS/(2^8)));
      | REGISTER_ADDRESS_LSB = uint8(rem(REGISTER_ADDRESS,2^8));
  wires:
  Constant1/1 -> I2C WRITE: SYSRANGE_START/1(DATA)

== system CAR_CONTROL_SYSTEM/HARDWARE/SENSORS/WALL RANGE SENSOR/VL6180X_I2C_REAR/VL6180X INITIALIZATION/CHECK INITIALIZATION ==
  Compare To Constant1 : simulink/Logic and Bit Operations/Compare To Constant  relop===  const=hex2dec('1F')  OutDataTypeStr=boolean
  Compare To Constant2 : simulink/Logic and Bit Operations/Compare To Constant  relop===  const=hex2dec('31')  OutDataTypeStr=boolean
  Compare To Constant3 : simulink/Logic and Bit Operations/Compare To Constant  relop===  const=hex2dec('00')  OutDataTypeStr=boolean
  Compare To Constant4 : simulink/Logic and Bit Operations/Compare To Constant  relop===  const=hex2dec('63')  OutDataTypeStr=boolean
  Compare To Constant5 : simulink/Logic and Bit Operations/Compare To Constant  relop===  const=hex2dec('24')  OutDataTypeStr=boolean
  Demux : Demux  Outputs=2
  I2C READ: SYSALS_INTEGRATION_PERIOD : Subsystem  mask{SLAVE_ADDRESS=VL6180X.ADDRESS, REGISTER_ADDRESS=VL6180X.SYSALS_INTEGRATION_PERIOD, N=2}
      mask prompts: SLAVE_ADDRESS "SLAVE ADDRESS"; REGISTER_ADDRESS "REGISTER ADDRESS"; N "NUMBER OF DATA (bytes)"
  I2C READ: SYSRANGE_MAX_CONVERGENCE_TIME : Subsystem  mask{SLAVE_ADDRESS=VL6180X.ADDRESS, REGISTER_ADDRESS=VL6180X.SYSRANGE_MAX_CONVERGENCE_TIME, N=1}
      mask prompts: SLAVE_ADDRESS "SLAVE ADDRESS"; REGISTER_ADDRESS "REGISTER ADDRESS"; N "NUMBER OF DATA (bytes)"
  "I2C READ: 0x1A7 " : Subsystem  mask{SLAVE_ADDRESS=VL6180X.ADDRESS, REGISTER_ADDRESS=hex2dec('1A7'), N=1}
      mask prompts: SLAVE_ADDRESS "SLAVE ADDRESS"; REGISTER_ADDRESS "REGISTER ADDRESS"; N "NUMBER OF DATA (bytes)"
  I2C WRITE: SYSTEM_INTERRUPT_CONFIG_GPIO : Subsystem  mask{SLAVE_ADDRESS=VL6180X.ADDRESS, REGISTER_ADDRESS=VL6180X.SYSTEM_INTERRUPT_CONFIG_GPIO, N=1}
      mask prompts: SLAVE_ADDRESS "SLAVE ADDRESS"; REGISTER_ADDRESS "REGISTER ADDRESS"; N "NUMBER OF DATA (bytes)"
  Logical Operator : Logic  Inputs=5  IconShape=distinctive  AllPortsSameDT=off  OutDataTypeStr=boolean
  STATUS : Outport  VectorParamsAs1DForOutWhenUnconnected=off
  wires:
  Logical Operator/1 -> STATUS/1
  Compare To Constant3/1 -> Logical Operator/2
  Compare To Constant4/1 -> Logical Operator/3
  Compare To Constant1/1 -> Logical Operator/1
  Compare To Constant5/1 -> Logical Operator/4
  I2C WRITE: SYSTEM_INTERRUPT_CONFIG_GPIO/1(DATA) -> Compare To Constant5/1
  I2C READ: SYSALS_INTEGRATION_PERIOD/1(DATA) -> Demux/1
  I2C READ: SYSRANGE_MAX_CONVERGENCE_TIME/1(DATA) -> Compare To Constant2/1
  Demux/1 -> Compare To Constant3/1
  Compare To Constant2/1 -> Logical Operator/5
  "I2C READ: 0x1A7 "/1(DATA) -> Compare To Constant1/1
  Demux/2 -> Compare To Constant4/1

== system CAR_CONTROL_SYSTEM/HARDWARE/SENSORS/WALL RANGE SENSOR/VL6180X_I2C_REAR/VL6180X INITIALIZATION/I2C READ: SYSTEM_FRESH_OUT_OF_RESET ==
  Constant : Constant  Value=REGISTER_ADDRESS  OutDataTypeStr=uint16  SampleTime=SAMPLING_TIME
  DATA TO BE READ : raspberrypiCommlib/I2C Controller Read  Priority=20  BoardProperty=Pi 3 Model B+  I2CModule=1  Mode=Master  SlaveAddress=SLAVE_ADDRESS  SlaveByteOrder=BigEndian  Direction=Receiver  RegisterAddressMode=off  RegisterAddress=0  SlaveDataType=uint8  DataLength=uint8(N)  NoAck=off  RepeatedStart=off  OutputStatus=off  SampleTime=SAMPLING_TIME
  REGISTER ADDRESS : raspberrypiCommlib/I2C Controller Write  Priority=10  BoardProperty=Pi 3 Model B+  I2CModule=1  Mode=Master  SlaveAddress=SLAVE_ADDRESS  SlaveByteOrder=BigEndian  Direction=Transmitter  RegisterAddressMode=off  RegisterAddress=hex2dec('207')  SlaveDataType=uint8  DataLength=1  NoAck=off  RepeatedStart=off  OutputStatus=off
  DATA : Outport  VectorParamsAs1DForOutWhenUnconnected=off
  wires:
  DATA TO BE READ/1 -> DATA/1
  Constant/1 -> REGISTER ADDRESS/1

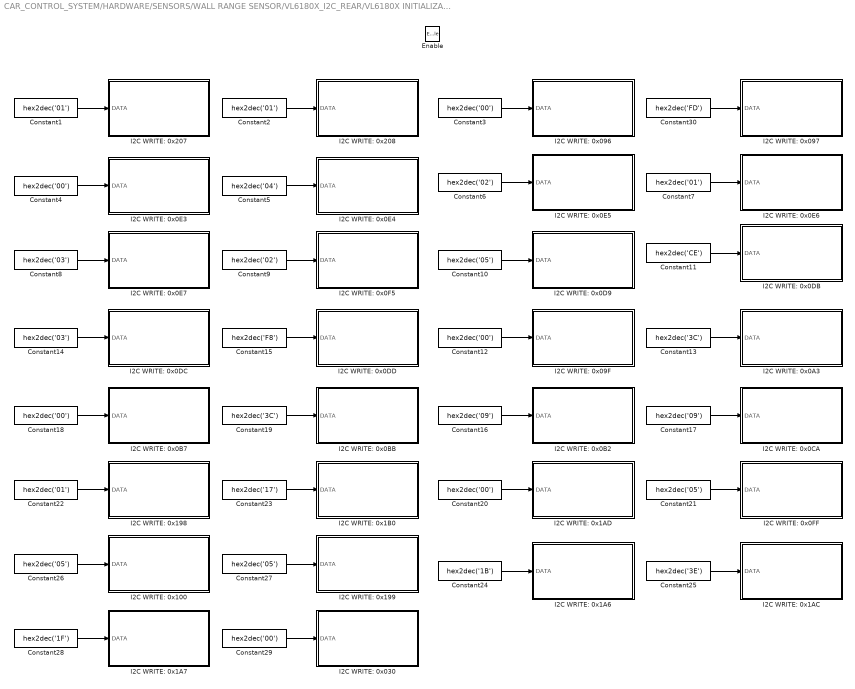
== system CAR_CONTROL_SYSTEM/HARDWARE/SENSORS/WALL RANGE SENSOR/VL6180X_I2C_REAR/VL6180X INITIALIZATION/LOAD PRIVATE REGISTERS (MANDATORY) ==
  Enable : EnablePort
  Constant{1..2,7,22} (4 alike) : Constant  Value=hex2dec('01')  OutDataTypeStr=uint8  SampleTime=SAMPLING_TIME
  Constant{10,21,26..27} (4 alike) : Constant  Value=hex2dec('05')  OutDataTypeStr=uint8  SampleTime=SAMPLING_TIME
  Constant11 : Constant  Value=hex2dec('CE')  OutDataTypeStr=uint8  SampleTime=SAMPLING_TIME
  Constant{3..4,12,18,20,29} (6 alike) : Constant  Value=hex2dec('00')  OutDataTypeStr=uint8  SampleTime=SAMPLING_TIME
  Constant13 : Constant  Value=hex2dec('3C')  OutDataTypeStr=uint8  SampleTime=SAMPLING_TIME
  Constant14 : Constant  Value=hex2dec('03')  OutDataTypeStr=uint8  SampleTime=SAMPLING_TIME
  Constant15 : Constant  Value=hex2dec('F8')  OutDataTypeStr=uint8  SampleTime=SAMPLING_TIME
  Constant16 : Constant  Value=hex2dec('09')  OutDataTypeStr=uint8  SampleTime=SAMPLING_TIME
  Constant17 : Constant  Value=hex2dec('09')  OutDataTypeStr=uint8  SampleTime=SAMPLING_TIME
  Constant19 : Constant  Value=hex2dec('3C')  OutDataTypeStr=uint8  SampleTime=SAMPLING_TIME
  Constant23 : Constant  Value=hex2dec('17')  OutDataTypeStr=uint8  SampleTime=SAMPLING_TIME
  Constant24 : Constant  Value=hex2dec('1B')  OutDataTypeStr=uint8  SampleTime=SAMPLING_TIME
  Constant25 : Constant  Value=hex2dec('3E')  OutDataTypeStr=uint8  SampleTime=SAMPLING_TIME
  Constant28 : Constant  Value=hex2dec('1F')  OutDataTypeStr=uint8  SampleTime=SAMPLING_TIME
  Constant30 : Constant  Value=hex2dec('FD')  OutDataTypeStr=uint8  SampleTime=SAMPLING_TIME
  Constant5 : Constant  Value=hex2dec('04')  OutDataTypeStr=uint8  SampleTime=SAMPLING_TIME
  Constant6 : Constant  Value=hex2dec('02')  OutDataTypeStr=uint8  SampleTime=SAMPLING_TIME
  Constant8 : Constant  Value=hex2dec('03')  OutDataTypeStr=uint8  SampleTime=SAMPLING_TIME
  Constant9 : Constant  Value=hex2dec('02')  OutDataTypeStr=uint8  SampleTime=SAMPLING_TIME
  "I2C WRITE: 0x030 " : Subsystem  mask{SLAVE_ADDRESS=VL6180X.ADDRESS, REGISTER_ADDRESS=hex2dec('030')}
      mask prompts: SLAVE_ADDRESS "SLAVE ADDRESS"; REGISTER_ADDRESS "REGISTER ADDRESS"
      mask init:
      | REGISTER_ADDRESS_MSB = uint8(floor(REGISTER_ADDRESS/(2^8)));
      | REGISTER_ADDRESS_LSB = uint8(rem(REGISTER_ADDRESS,2^8));
  I2C WRITE: 0x096 : Subsystem  mask{SLAVE_ADDRESS=VL6180X.ADDRESS, REGISTER_ADDRESS=hex2dec('096')}
      mask prompts: SLAVE_ADDRESS "SLAVE ADDRESS"; REGISTER_ADDRESS "REGISTER ADDRESS"
      mask init:
      | REGISTER_ADDRESS_MSB = uint8(floor(REGISTER_ADDRESS/(2^8)));
      | REGISTER_ADDRESS_LSB = uint8(rem(REGISTER_ADDRESS,2^8));
  I2C WRITE: 0x097 : Subsystem  mask{SLAVE_ADDRESS=VL6180X.ADDRESS, REGISTER_ADDRESS=hex2dec('097')}
      mask prompts: SLAVE_ADDRESS "SLAVE ADDRESS"; REGISTER_ADDRESS "REGISTER ADDRESS"
      mask init:
      | REGISTER_ADDRESS_MSB = uint8(floor(REGISTER_ADDRESS/(2^8)));
      | REGISTER_ADDRESS_LSB = uint8(rem(REGISTER_ADDRESS,2^8));
  I2C WRITE: 0x09F : Subsystem  mask{SLAVE_ADDRESS=VL6180X.ADDRESS, REGISTER_ADDRESS=hex2dec('09F')}
      mask prompts: SLAVE_ADDRESS "SLAVE ADDRESS"; REGISTER_ADDRESS "REGISTER ADDRESS"
      mask init:
      | REGISTER_ADDRESS_MSB = uint8(floor(REGISTER_ADDRESS/(2^8)));
      | REGISTER_ADDRESS_LSB = uint8(rem(REGISTER_ADDRESS,2^8));
  I2C WRITE: 0x0A3 : Subsystem  mask{SLAVE_ADDRESS=VL6180X.ADDRESS, REGISTER_ADDRESS=hex2dec('0A3')}
      mask prompts: SLAVE_ADDRESS "SLAVE ADDRESS"; REGISTER_ADDRESS "REGISTER ADDRESS"
      mask init:
      | REGISTER_ADDRESS_MSB = uint8(floor(REGISTER_ADDRESS/(2^8)));
      | REGISTER_ADDRESS_LSB = uint8(rem(REGISTER_ADDRESS,2^8));
  I2C WRITE: 0x0B2 : Subsystem  mask{SLAVE_ADDRESS=VL6180X.ADDRESS, REGISTER_ADDRESS=hex2dec('0B2')}
      mask prompts: SLAVE_ADDRESS "SLAVE ADDRESS"; REGISTER_ADDRESS "REGISTER ADDRESS"
      mask init:
      | REGISTER_ADDRESS_MSB = uint8(floor(REGISTER_ADDRESS/(2^8)));
      | REGISTER_ADDRESS_LSB = uint8(rem(REGISTER_ADDRESS,2^8));
  I2C WRITE: 0x0B7 : Subsystem  mask{SLAVE_ADDRESS=VL6180X.ADDRESS, REGISTER_ADDRESS=hex2dec('0B7')}
      mask prompts: SLAVE_ADDRESS "SLAVE ADDRESS"; REGISTER_ADDRESS "REGISTER ADDRESS"
      mask init:
      | REGISTER_ADDRESS_MSB = uint8(floor(REGISTER_ADDRESS/(2^8)));
      | REGISTER_ADDRESS_LSB = uint8(rem(REGISTER_ADDRESS,2^8));
  I2C WRITE: 0x0BB : Subsystem  mask{SLAVE_ADDRESS=VL6180X.ADDRESS, REGISTER_ADDRESS=hex2dec('0BB')}
      mask prompts: SLAVE_ADDRESS "SLAVE ADDRESS"; REGISTER_ADDRESS "REGISTER ADDRESS"
      mask init:
      | REGISTER_ADDRESS_MSB = uint8(floor(REGISTER_ADDRESS/(2^8)));
      | REGISTER_ADDRESS_LSB = uint8(rem(REGISTER_ADDRESS,2^8));
  I2C WRITE: 0x0CA : Subsystem  mask{SLAVE_ADDRESS=VL6180X.ADDRESS, REGISTER_ADDRESS=hex2dec('0CA')}
      mask prompts: SLAVE_ADDRESS "SLAVE ADDRESS"; REGISTER_ADDRESS "REGISTER ADDRESS"
      mask init:
      | REGISTER_ADDRESS_MSB = uint8(floor(REGISTER_ADDRESS/(2^8)));
      | REGISTER_ADDRESS_LSB = uint8(rem(REGISTER_ADDRESS,2^8));
  I2C WRITE: 0x0D9 : Subsystem  mask{SLAVE_ADDRESS=VL6180X.ADDRESS, REGISTER_ADDRESS=hex2dec('0D9')}
      mask prompts: SLAVE_ADDRESS "SLAVE ADDRESS"; REGISTER_ADDRESS "REGISTER ADDRESS"
      mask init:
      | REGISTER_ADDRESS_MSB = uint8(floor(REGISTER_ADDRESS/(2^8)));
      | REGISTER_ADDRESS_LSB = uint8(rem(REGISTER_ADDRESS,2^8));
  I2C WRITE: 0x0DB : Subsystem  mask{SLAVE_ADDRESS=VL6180X.ADDRESS, REGISTER_ADDRESS=hex2dec('0DB')}
      mask prompts: SLAVE_ADDRESS "SLAVE ADDRESS"; REGISTER_ADDRESS "REGISTER ADDRESS"
      mask init:
      | REGISTER_ADDRESS_MSB = uint8(floor(REGISTER_ADDRESS/(2^8)));
      | REGISTER_ADDRESS_LSB = uint8(rem(REGISTER_ADDRESS,2^8));
  I2C WRITE: 0x0DC : Subsystem  mask{SLAVE_ADDRESS=VL6180X.ADDRESS, REGISTER_ADDRESS=hex2dec('0DB')}
      mask prompts: SLAVE_ADDRESS "SLAVE ADDRESS"; REGISTER_ADDRESS "REGISTER ADDRESS"
      mask init:
      | REGISTER_ADDRESS_MSB = uint8(floor(REGISTER_ADDRESS/(2^8)));
      | REGISTER_ADDRESS_LSB = uint8(rem(REGISTER_ADDRESS,2^8));
  I2C WRITE: 0x0DD : Subsystem  mask{SLAVE_ADDRESS=VL6180X.ADDRESS, REGISTER_ADDRESS=hex2dec('0DD')}
      mask prompts: SLAVE_ADDRESS "SLAVE ADDRESS"; REGISTER_ADDRESS "REGISTER ADDRESS"
      mask init:
      | REGISTER_ADDRESS_MSB = uint8(floor(REGISTER_ADDRESS/(2^8)));
      | REGISTER_ADDRESS_LSB = uint8(rem(REGISTER_ADDRESS,2^8));
  I2C WRITE: 0x0E3 : Subsystem  mask{SLAVE_ADDRESS=VL6180X.ADDRESS, REGISTER_ADDRESS=hex2dec('0E3')}
      mask prompts: SLAVE_ADDRESS "SLAVE ADDRESS"; REGISTER_ADDRESS "REGISTER ADDRESS"
      mask init:
      | REGISTER_ADDRESS_MSB = uint8(floor(REGISTER_ADDRESS/(2^8)));
      | REGISTER_ADDRESS_LSB = uint8(rem(REGISTER_ADDRESS,2^8));
  I2C WRITE: 0x0E4 : Subsystem  mask{SLAVE_ADDRESS=VL6180X.ADDRESS, REGISTER_ADDRESS=hex2dec('0E4')}
      mask prompts: SLAVE_ADDRESS "SLAVE ADDRESS"; REGISTER_ADDRESS "REGISTER ADDRESS"
      mask init:
      | REGISTER_ADDRESS_MSB = uint8(floor(REGISTER_ADDRESS/(2^8)));
      | REGISTER_ADDRESS_LSB = uint8(rem(REGISTER_ADDRESS,2^8));
  I2C WRITE: 0x0E5 : Subsystem  mask{SLAVE_ADDRESS=VL6180X.ADDRESS, REGISTER_ADDRESS=hex2dec('0E5')}
      mask prompts: SLAVE_ADDRESS "SLAVE ADDRESS"; REGISTER_ADDRESS "REGISTER ADDRESS"
      mask init:
      | REGISTER_ADDRESS_MSB = uint8(floor(REGISTER_ADDRESS/(2^8)));
      | REGISTER_ADDRESS_LSB = uint8(rem(REGISTER_ADDRESS,2^8));
  I2C WRITE: 0x0E6 : Subsystem  mask{SLAVE_ADDRESS=VL6180X.ADDRESS, REGISTER_ADDRESS=hex2dec('0E6')}
      mask prompts: SLAVE_ADDRESS "SLAVE ADDRESS"; REGISTER_ADDRESS "REGISTER ADDRESS"
      mask init:
      | REGISTER_ADDRESS_MSB = uint8(floor(REGISTER_ADDRESS/(2^8)));
      | REGISTER_ADDRESS_LSB = uint8(rem(REGISTER_ADDRESS,2^8));
  I2C WRITE: 0x0E7 : Subsystem  mask{SLAVE_ADDRESS=VL6180X.ADDRESS, REGISTER_ADDRESS=hex2dec('0E7')}
      mask prompts: SLAVE_ADDRESS "SLAVE ADDRESS"; REGISTER_ADDRESS "REGISTER ADDRESS"
      mask init:
      | REGISTER_ADDRESS_MSB = uint8(floor(REGISTER_ADDRESS/(2^8)));
      | REGISTER_ADDRESS_LSB = uint8(rem(REGISTER_ADDRESS,2^8));
  I2C WRITE: 0x0F5 : Subsystem  mask{SLAVE_ADDRESS=VL6180X.ADDRESS, REGISTER_ADDRESS=hex2dec('0F5')}
      mask prompts: SLAVE_ADDRESS "SLAVE ADDRESS"; REGISTER_ADDRESS "REGISTER ADDRESS"
      mask init:
      | REGISTER_ADDRESS_MSB = uint8(floor(REGISTER_ADDRESS/(2^8)));
      | REGISTER_ADDRESS_LSB = uint8(rem(REGISTER_ADDRESS,2^8));
  "I2C WRITE: 0x0FF " : Subsystem  mask{SLAVE_ADDRESS=VL6180X.ADDRESS, REGISTER_ADDRESS=hex2dec('0FF')}
      mask prompts: SLAVE_ADDRESS "SLAVE ADDRESS"; REGISTER_ADDRESS "REGISTER ADDRESS"
      mask init:
      | REGISTER_ADDRESS_MSB = uint8(floor(REGISTER_ADDRESS/(2^8)));
      | REGISTER_ADDRESS_LSB = uint8(rem(REGISTER_ADDRESS,2^8));
  "I2C WRITE: 0x100 " : Subsystem  mask{SLAVE_ADDRESS=VL6180X.ADDRESS, REGISTER_ADDRESS=hex2dec('100')}
      mask prompts: SLAVE_ADDRESS "SLAVE ADDRESS"; REGISTER_ADDRESS "REGISTER ADDRESS"
      mask init:
      | REGISTER_ADDRESS_MSB = uint8(floor(REGISTER_ADDRESS/(2^8)));
      | REGISTER_ADDRESS_LSB = uint8(rem(REGISTER_ADDRESS,2^8));
  I2C WRITE: 0x198 : Subsystem  mask{SLAVE_ADDRESS=VL6180X.ADDRESS, REGISTER_ADDRESS=hex2dec('198')}
      mask prompts: SLAVE_ADDRESS "SLAVE ADDRESS"; REGISTER_ADDRESS "REGISTER ADDRESS"
      mask init:
      | REGISTER_ADDRESS_MSB = uint8(floor(REGISTER_ADDRESS/(2^8)));
      | REGISTER_ADDRESS_LSB = uint8(rem(REGISTER_ADDRESS,2^8));
  "I2C WRITE: 0x199 " : Subsystem  mask{SLAVE_ADDRESS=VL6180X.ADDRESS, REGISTER_ADDRESS=hex2dec('199')}
      mask prompts: SLAVE_ADDRESS "SLAVE ADDRESS"; REGISTER_ADDRESS "REGISTER ADDRESS"
      mask init:
      | REGISTER_ADDRESS_MSB = uint8(floor(REGISTER_ADDRESS/(2^8)));
      | REGISTER_ADDRESS_LSB = uint8(rem(REGISTER_ADDRESS,2^8));
  "I2C WRITE: 0x1A6 " : Subsystem  mask{SLAVE_ADDRESS=VL6180X.ADDRESS, REGISTER_ADDRESS=hex2dec('1A6')}
      mask prompts: SLAVE_ADDRESS "SLAVE ADDRESS"; REGISTER_ADDRESS "REGISTER ADDRESS"
      mask init:
      | REGISTER_ADDRESS_MSB = uint8(floor(REGISTER_ADDRESS/(2^8)));
      | REGISTER_ADDRESS_LSB = uint8(rem(REGISTER_ADDRESS,2^8));
  "I2C WRITE: 0x1A7 " : Subsystem  mask{SLAVE_ADDRESS=VL6180X.ADDRESS, REGISTER_ADDRESS=hex2dec('1A7')}
      mask prompts: SLAVE_ADDRESS "SLAVE ADDRESS"; REGISTER_ADDRESS "REGISTER ADDRESS"
      mask init:
      | REGISTER_ADDRESS_MSB = uint8(floor(REGISTER_ADDRESS/(2^8)));
      | REGISTER_ADDRESS_LSB = uint8(rem(REGISTER_ADDRESS,2^8));
  "I2C WRITE: 0x1AC " : Subsystem  mask{SLAVE_ADDRESS=VL6180X.ADDRESS, REGISTER_ADDRESS=hex2dec('1AC')}
      mask prompts: SLAVE_ADDRESS "SLAVE ADDRESS"; REGISTER_ADDRESS "REGISTER ADDRESS"
      mask init:
      | REGISTER_ADDRESS_MSB = uint8(floor(REGISTER_ADDRESS/(2^8)));
      | REGISTER_ADDRESS_LSB = uint8(rem(REGISTER_ADDRESS,2^8));
  "I2C WRITE: 0x1AD " : Subsystem  mask{SLAVE_ADDRESS=VL6180X.ADDRESS, REGISTER_ADDRESS=hex2dec('1AD')}
      mask prompts: SLAVE_ADDRESS "SLAVE ADDRESS"; REGISTER_ADDRESS "REGISTER ADDRESS"
      mask init:
      | REGISTER_ADDRESS_MSB = uint8(floor(REGISTER_ADDRESS/(2^8)));
      | REGISTER_ADDRESS_LSB = uint8(rem(REGISTER_ADDRESS,2^8));
  "I2C WRITE: 0x1B0 " : Subsystem  mask{SLAVE_ADDRESS=VL6180X.ADDRESS, REGISTER_ADDRESS=hex2dec('1B0')}
      mask prompts: SLAVE_ADDRESS "SLAVE ADDRESS"; REGISTER_ADDRESS "REGISTER ADDRESS"
      mask init:
      | REGISTER_ADDRESS_MSB = uint8(floor(REGISTER_ADDRESS/(2^8)));
      | REGISTER_ADDRESS_LSB = uint8(rem(REGISTER_ADDRESS,2^8));
  I2C WRITE: 0x207 : Subsystem  mask{SLAVE_ADDRESS=VL6180X.ADDRESS, REGISTER_ADDRESS=hex2dec('207')}
      mask prompts: SLAVE_ADDRESS "SLAVE ADDRESS"; REGISTER_ADDRESS "REGISTER ADDRESS"
      mask init:
      | REGISTER_ADDRESS_MSB = uint8(floor(REGISTER_ADDRESS/(2^8)));
      | REGISTER_ADDRESS_LSB = uint8(rem(REGISTER_ADDRESS,2^8));
  I2C WRITE: 0x208 : Subsystem  mask{SLAVE_ADDRESS=VL6180X.ADDRESS, REGISTER_ADDRESS=hex2dec('208')}
      mask prompts: SLAVE_ADDRESS "SLAVE ADDRESS"; REGISTER_ADDRESS "REGISTER ADDRESS"
      mask init:
      | REGISTER_ADDRESS_MSB = uint8(floor(REGISTER_ADDRESS/(2^8)));
      | REGISTER_ADDRESS_LSB = uint8(rem(REGISTER_ADDRESS,2^8));
  wires:
  Constant29/1 -> "I2C WRITE: 0x030 "/1(DATA)
  Constant28/1 -> "I2C WRITE: 0x1A7 "/1(DATA)
  Constant25/1 -> "I2C WRITE: 0x1AC "/1(DATA)
  Constant24/1 -> "I2C WRITE: 0x1A6 "/1(DATA)
  Constant27/1 -> "I2C WRITE: 0x199 "/1(DATA)
  Constant26/1 -> "I2C WRITE: 0x100 "/1(DATA)
  Constant21/1 -> "I2C WRITE: 0x0FF "/1(DATA)
  Constant20/1 -> "I2C WRITE: 0x1AD "/1(DATA)
  Constant23/1 -> "I2C WRITE: 0x1B0 "/1(DATA)
  Constant22/1 -> I2C WRITE: 0x198/1(DATA)
  Constant17/1 -> I2C WRITE: 0x0CA/1(DATA)
  Constant16/1 -> I2C WRITE: 0x0B2/1(DATA)
  Constant19/1 -> I2C WRITE: 0x0BB/1(DATA)
  Constant18/1 -> I2C WRITE: 0x0B7/1(DATA)
  Constant13/1 -> I2C WRITE: 0x0A3/1(DATA)
  Constant12/1 -> I2C WRITE: 0x09F/1(DATA)
  Constant15/1 -> I2C WRITE: 0x0DD/1(DATA)
  Constant14/1 -> I2C WRITE: 0x0DC/1(DATA)
  Constant11/1 -> I2C WRITE: 0x0DB/1(DATA)
  Constant10/1 -> I2C WRITE: 0x0D9/1(DATA)
  Constant9/1 -> I2C WRITE: 0x0F5/1(DATA)
  Constant8/1 -> I2C WRITE: 0x0E7/1(DATA)
  Constant7/1 -> I2C WRITE: 0x0E6/1(DATA)
  Constant6/1 -> I2C WRITE: 0x0E5/1(DATA)
  Constant5/1 -> I2C WRITE: 0x0E4/1(DATA)
  Constant4/1 -> I2C WRITE: 0x0E3/1(DATA)
  Constant30/1 -> I2C WRITE: 0x097/1(DATA)
  Constant3/1 -> I2C WRITE: 0x096/1(DATA)
  Constant2/1 -> I2C WRITE: 0x208/1(DATA)
  Constant1/1 -> I2C WRITE: 0x207/1(DATA)

== system CAR_CONTROL_SYSTEM/HARDWARE/SENSORS/WALL RANGE SENSOR/VL6180X_I2C_REAR/VL6180X INITIALIZATION/LOAD PUBLIC REGISTERS (OPTIONAL) ==
  note: sysrange__intermeasurement_period = 1 (20 ms)
  note: sysals__intermeasurement_period = 49 (500 ms)
  note: als_int_mode = 4 (ALS new sample ready interrupt);
      | range_int_mode = 4 (range new sample ready interrupt)
  Enable : EnablePort
  Constant2 : Constant  Value=VL6180X.SYSRANGE_INTERMEASUREMENT_PERIOD_BYTE  OutDataTypeStr=uint8  SampleTime=SAMPLING_TIME
  Constant3 : Constant  Value=hex2dec('24')  OutDataTypeStr=uint8  SampleTime=SAMPLING_TIME
  Constant4 : Constant  Commented=on  Value=VL6180X.SYSALS_INTERMEASUREMENT_PERIOD_BYTE  OutDataTypeStr=uint8  SampleTime=SAMPLING_TIME
  I2C WRITE: SYSRANGE_INTERMEASUREMENT_PERIOD : Subsystem  mask{SLAVE_ADDRESS=VL6180X.ADDRESS, REGISTER_ADDRESS=VL6180X.SYSRANGE_INTERMEASUREMENT_PERIOD}
      mask prompts: SLAVE_ADDRESS "SLAVE ADDRESS"; REGISTER_ADDRESS "REGISTER ADDRESS"
      mask init:
      | REGISTER_ADDRESS_MSB = uint8(floor(REGISTER_ADDRESS/(2^8)));
      | REGISTER_ADDRESS_LSB = uint8(rem(REGISTER_ADDRESS,2^8));
  I2C WRITE: SYSALS_INTERMEASUREMENT_PERIOD : Subsystem  Commented=on  mask{SLAVE_ADDRESS=VL6180X.ADDRESS, REGISTER_ADDRESS=VL6180X.SYSALS_INTERMEASUREMENT_PERIOD}
      mask prompts: SLAVE_ADDRESS "SLAVE ADDRESS"; REGISTER_ADDRESS "REGISTER ADDRESS"
      mask init:
      | REGISTER_ADDRESS_MSB = uint8(floor(REGISTER_ADDRESS/(2^8)));
      | REGISTER_ADDRESS_LSB = uint8(rem(REGISTER_ADDRESS,2^8));
  I2C WRITE: SYSTEM_INTERRUPT_CONFIG_GPIO : Subsystem  mask{SLAVE_ADDRESS=VL6180X.ADDRESS, REGISTER_ADDRESS=VL6180X.SYSTEM_INTERRUPT_CONFIG_GPIO}
      mask prompts: SLAVE_ADDRESS "SLAVE ADDRESS"; REGISTER_ADDRESS "REGISTER ADDRESS"
      mask init:
      | REGISTER_ADDRESS_MSB = uint8(floor(REGISTER_ADDRESS/(2^8)));
      | REGISTER_ADDRESS_LSB = uint8(rem(REGISTER_ADDRESS,2^8));
  wires:
  Constant2/1 -> I2C WRITE: SYSRANGE_INTERMEASUREMENT_PERIOD/1(DATA)
  Constant3/1 -> I2C WRITE: SYSTEM_INTERRUPT_CONFIG_GPIO/1(DATA)
  Constant4/1 -> I2C WRITE: SYSALS_INTERMEASUREMENT_PERIOD/1(DATA)
